simulink subsystem "ScanDc"  (R2025a)
settings: Solver=VariableStepAuto  StartTime=0.0  StopTime=10.0  RelTol=1e-3
model mask{F0=0, Theta0=0, Kp_LF=0, Ki_LF=0, Ts=0, Amplitudedc=scan.Vdc, Amplitude=0, Amplitude1=0, voltagedc=HVDC.Vdc, voltage=0, mva=0, f=scan.f, Tdis=scan.start, Tend=scan.end, T=1/scan.samplingfrequency}
  mask prompts: F0 "Initial frequency (Hz)"; Theta0 "Inital angle (deg)"; Kp_LF "Proportional gain"; Ki_LF "Integral gain"; Ts "Sample time (sec)"; Amplitudedc "DC voltage disturbance (PU)"; Amplitude "D axis voltage disturbance (PU)"; Amplitude1 "Q axis voltage disturbance (PU)"; voltagedc "Base DC Voltage (V)"; voltage "Base AC Voltage (V)"; mva "Base voltr ampere (VA)"; f "Disturbance Frequency (Hz)"; Tdis "Disturbance start time (sec)"; Tend "Disturbance end time (sec)"; T "Sample Time of PRBS (sec)"
undefined symbols (not defined in the file): DiscIntNeverNeededParam, ee_sli_rtmsupport, gcbh, w
libraries: slctrl_fre x6, eeGeneralControl x4, slctrl_signal x3, eeTransforms x2, ee_lib x1, nesl_utility x1, simulink x1
(part 2 of 2)

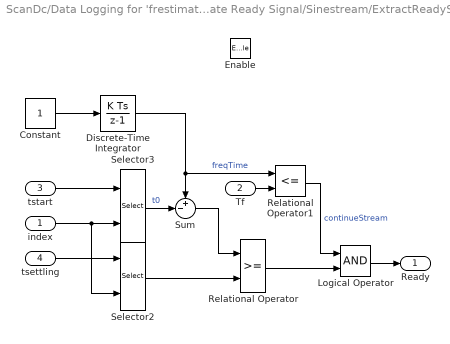
== system ScanDc/Data Logging for 'frestimate'2/Generate Ready Signal/Sinestream/ExtractReadySignal/Triggered Subsystem ==
  index : Inport
  Tf : Inport  Port=2
  tstart : Inport  Port=3
  tsettling : Inport  Port=4
  Enable : EnablePort
  Constant : Constant  OutDataTypeStr=double
  Discrete-Time Integrator : DiscreteIntegrator  SampleTime=Ts  ICPrevOutput=DiscIntNeverNeededParam  ICPrevScaledInput=DiscIntNeverNeededParam
  Logical Operator : Logic  AllPortsSameDT=off  OutDataTypeStr=boolean
  Relational Operator : RelationalOperator  OutDataTypeStr=boolean  RndMeth=Simplest  InputSameDT=off
  Relational Operator1 : RelationalOperator  Operator=<=  OutDataTypeStr=boolean  RndMeth=Simplest  InputSameDT=off
  Selector2 : Selector  InputPortWidth=nw  IndexOptions=Index vector (port)  Indices=[1 3]  OutputSizes=1
  Selector3 : Selector  InputPortWidth=nw  IndexOptions=Index vector (port)  Indices=[1 3]  OutputSizes=1
  Sum : Sum  Inputs=+-|
  Ready : Outport
  wires:
  Logical Operator/1 -> Ready/1
  Relational Operator1/1 -> Logical Operator/1  "continueStream"
  Tf/1 -> Relational Operator1/2
  Relational Operator/1 -> Logical Operator/2
  index/1 -> Selector3/2, Selector2/2
  Discrete-Time Integrator/1 -> Relational Operator1/1, Sum/1  "freqTime"
  Selector3/1 -> Sum/2  "t0"
  Selector2/1 -> Relational Operator/2
  tsettling/1 -> Selector2/1
  tstart/1 -> Selector3/1
  Sum/1 -> Relational Operator/1
  Constant/1 -> Discrete-Time Integrator/1

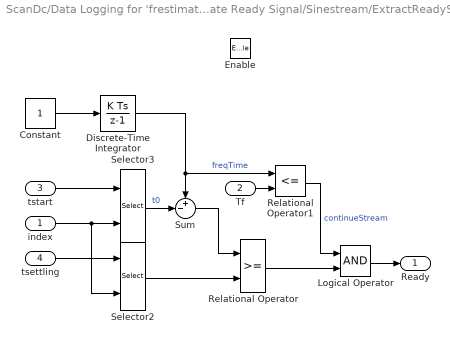
== system ScanDc/Data Logging for 'frestimate'3/Generate Ready Signal/Sinestream/ExtractReadySignal/Triggered Subsystem ==
  index : Inport
  Tf : Inport  Port=2
  tstart : Inport  Port=3
  tsettling : Inport  Port=4
  Enable : EnablePort
  Constant : Constant  OutDataTypeStr=double
  Discrete-Time Integrator : DiscreteIntegrator  SampleTime=Ts  ICPrevOutput=DiscIntNeverNeededParam  ICPrevScaledInput=DiscIntNeverNeededParam
  Logical Operator : Logic  AllPortsSameDT=off  OutDataTypeStr=boolean
  Relational Operator : RelationalOperator  OutDataTypeStr=boolean  RndMeth=Simplest  InputSameDT=off
  Relational Operator1 : RelationalOperator  Operator=<=  OutDataTypeStr=boolean  RndMeth=Simplest  InputSameDT=off
  Selector2 : Selector  InputPortWidth=nw  IndexOptions=Index vector (port)  Indices=[1 3]  OutputSizes=1
  Selector3 : Selector  InputPortWidth=nw  IndexOptions=Index vector (port)  Indices=[1 3]  OutputSizes=1
  Sum : Sum  Inputs=+-|
  Ready : Outport
  wires:
  Logical Operator/1 -> Ready/1
  Relational Operator1/1 -> Logical Operator/1  "continueStream"
  Tf/1 -> Relational Operator1/2
  Relational Operator/1 -> Logical Operator/2
  index/1 -> Selector3/2, Selector2/2
  Discrete-Time Integrator/1 -> Relational Operator1/1, Sum/1  "freqTime"
  Selector3/1 -> Sum/2  "t0"
  Selector2/1 -> Relational Operator/2
  tsettling/1 -> Selector2/1
  tstart/1 -> Selector3/1
  Sum/1 -> Relational Operator/1
  Constant/1 -> Discrete-Time Integrator/1

== matlab function ScanDc/Data Logging for 'frestimate'1/Generate Ready Signal/Sinestream/ExtractReadySignal/MATLAB Function ==
  data: Frequencies input; Tf output; Ts input; NumOfEstPeriod input; NumOfSetPeriod input; tstart output; tsettling output
function [Tf, tstart, tsettling] = extractReadySignal(Frequencies,Ts,NumOfEstPeriod,NumOfSetPeriod)
% obtain the number of periods requested for each frequency
NumPeriods = NumOfEstPeriod + NumOfSetPeriod;
% obtain period time for each frequency
T = 2*pi./Frequencies;
% define experiment length for each frequency (add two samples for CA)
Length = NumPeriods.*T+2*Ts;
% calculate start time stamp for each frequency
CUMSUM = cumsum(Length);
tstart = [0;CUMSUM(1:end-1)];
% calculate the settling duration for each frequency (cannot be zero)
tsettling = [NumOfSetPeriod.*T];
% obtain the stop time for the experiment
Tf = CUMSUM(end);

== matlab function ScanDc/Data Logging for 'frestimate'2/Generate Ready Signal/Sinestream/ExtractReadySignal/MATLAB Function ==
  data: Frequencies input; Tf output; Ts input; NumOfEstPeriod input; NumOfSetPeriod input; tstart output; tsettling output
function [Tf, tstart, tsettling] = extractReadySignal(Frequencies,Ts,NumOfEstPeriod,NumOfSetPeriod)
% obtain the number of periods requested for each frequency
NumPeriods = NumOfEstPeriod + NumOfSetPeriod;
% obtain period time for each frequency
T = 2*pi./Frequencies;
% define experiment length for each frequency (add two samples for CA)
Length = NumPeriods.*T+2*Ts;
% calculate start time stamp for each frequency
CUMSUM = cumsum(Length);
tstart = [0;CUMSUM(1:end-1)];
% calculate the settling duration for each frequency (cannot be zero)
tsettling = [NumOfSetPeriod.*T];
% obtain the stop time for the experiment
Tf = CUMSUM(end);

== matlab function ScanDc/Data Logging for 'frestimate'3/Generate Ready Signal/Sinestream/ExtractReadySignal/MATLAB Function ==
  data: Frequencies input; Tf output; Ts input; NumOfEstPeriod input; NumOfSetPeriod input; tstart output; tsettling output
function [Tf, tstart, tsettling] = extractReadySignal(Frequencies,Ts,NumOfEstPeriod,NumOfSetPeriod)
% obtain the number of periods requested for each frequency
NumPeriods = NumOfEstPeriod + NumOfSetPeriod;
% obtain period time for each frequency
T = 2*pi./Frequencies;
% define experiment length for each frequency (add two samples for CA)
Length = NumPeriods.*T+2*Ts;
% calculate start time stamp for each frequency
CUMSUM = cumsum(Length);
tstart = [0;CUMSUM(1:end-1)];
% calculate the settling duration for each frequency (cannot be zero)
tsettling = [NumOfSetPeriod.*T];
% obtain the stop time for the experiment
Tf = CUMSUM(end);
